simulink model "E_Platoon"  (R2025b)
settings: Solver=FixedStepAuto  StartTime=0.0  StopTime=inf  FixedStep=0.1  RelTol=1e-3
values from neighbouring files (symbols this model uses):
  Battery_Capacity = [1,4500]    [EV_Truck.m]
  battery_SOC_resistance = battery_SOC(:,3)    [EV_Truck.m]
  battery_SOC_SOC = battery_SOC(:,1)    [EV_Truck.m]
  battery_SOC_voltage = battery_SOC(:,2)    [EV_Truck.m]
  motor_efficiency_efficiency = table2array(motor_efficiency(2:height(motor_efficiency),2:width(motor_efficiency)))    [EV_Truck.m]
  motor_efficiency_RPM = table2array(motor_efficiency(2:height(motor_efficiency),1))    [EV_Truck.m]
  motor_efficiency_torque = transpose(motor_efficiency_torque)    [EV_Truck.m]
  motor_RPM_torque = table2array(motor_torque(1:14,1))    [EV_Truck.m]
  motor_torque_RPM = table2array(motor_torque(1:14,2))    [EV_Truck.m]
undefined symbols (not defined in the file or in its folder): Battery_Initial_SOC, DiscIntNeverNeededParam
libraries: simulink x8, BatteryEstimators x4, mpcadaslib x2, slpidlib x2
(part 2 of 2)

== matlab function E_Platoon/FV2/Drag coefficient ==
  data: IVD input; C_drag output
function C_drag = fcn(IVD)
a = -0.4629;
b = -0.068;
c = 0.6441;

C_drag = a * exp(b * (IVD-8)) + c;

== matlab function E_Platoon/FV1/ACC system/MATLAB Function ==
  data: accel input; acceleration output
function acceleration  = fcn(accel)

if accel > 0 
    acceleration = (accel * 100)/0.15;
elseif accel < 0 
    acceleration = (accel * 100)/0.33;
else
    acceleration = 0; % accel이 0이거나 NaN일 경우에도 대응
end

== matlab function E_Platoon/FV1/Drag coefficient ==
  data: IVD input; C_drag output
function C_drag = fcn(IVD)
a = -0.4629;
b = -0.068;
c = 0.6441;

C_drag = a * exp(b * (IVD-8)) + c;

== matlab function E_Platoon/LV/MATLAB Function ==
  data: P input; OCV input; R0 input; I output
function I = current_from_power(P, OCV, R0)
% 1-R battery model:
%   Vt = OCV - R0*I
%   P  = Vt*I = I*(OCV - R0*I)
% => R0*I^2 - OCV*I + P = 0
%   I = (OCV - sqrt(OCV^2 - 4*R0*P)) / (2*R0)
%
%   P>0 -> I>0 (discharge)
%   P<0 -> I<0 (regen/charge)

epsR = 1e-12;
epsV = 1e-6;
R0  = max(R0, epsR);
OCV = max(OCV, epsV);

% Discriminant
D = OCV*OCV - 4*R0*P;

% If D < 0, the requested P is infeasible under this simple model.
% Clamp to 0 to avoid complex values (simple fallback).
if D < 0
    D = 0;
end

% Minus-branch current
I = (OCV - sqrt(D)) / (2*R0);

% Safety
if ~isfinite(I)
    I = 0;
end
end
